simulink model "tau_7_1"  (R2019b)
settings: Solver=VariableStepAuto  StartTime=0.0  StopTime=9  RelTol=1e-3
model workspace (MAT data in the model file):
  k = 0.5
libraries: slctrlblks x10, simulink x5
settings Model: Creator=Sergey  LastModifiedBy=Sergey

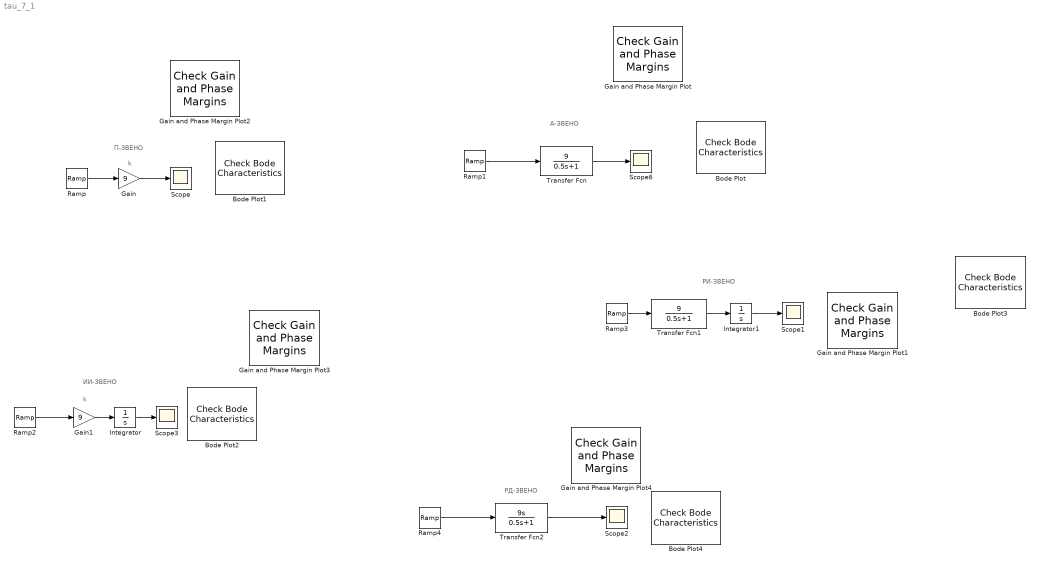
== system tau_7_1 ==
  note: РД-ЗВЕНО
  note: РИ-ЗВЕНО
  note: ИИ-ЗВЕНО
  note: А-ЗВЕНО
  note: П-ЗВЕНО
  note: k
  note: k
  Bode Plot : slctrlblks/Model Verification/Check Bode  Characteristics  InstantiateOnLoad=on  SaveOperatingPoints=off  LinearizationIOs={'/Ramp1', 1, 'in', 'off', '';'/Transfer Fcn', 1, 'out', 'off', ''}  LinearizeAt=SnapshotTimes  SnapshotTimes=[0]  TriggerType=rising  SampleTime=auto  RateConversionMethod=zoh  PreWarpFreq=10  UseExactDelayModel=off  UseFullBlockNameLabels=off  UseBusSignalLabels=off  enabled=on  stopWhenAssertionFail=off  export=off  ViewDlgPos=[1 41 1920 963]  OpenViewOnLoad=off  LaunchViewOnOpen=on  FrequencyUnits=rad/s  MagnitudeUnits=dB  PhaseUnits=deg  TimeUnits=seconds  EnableUpperBound=off  UpperBoundFrequencies=[]  UpperBoundMagnitudes=[]  EnableLowerBound=off  LowerBoundFrequencies=[]  LowerBoundMagnitudes=[]
      settings: SourceProductName=Simulink Control Design
  Bode Plot1 : slctrlblks/Model Verification/Check Bode  Characteristics  InstantiateOnLoad=on  SaveOperatingPoints=off  LinearizationIOs={'/Ramp', 1, 'in', 'off', '';'/Gain', 1, 'out', 'off', ''}  LinearizeAt=SnapshotTimes  SnapshotTimes=[0]  TriggerType=rising  SampleTime=auto  RateConversionMethod=zoh  PreWarpFreq=10  UseExactDelayModel=off  UseFullBlockNameLabels=off  UseBusSignalLabels=off  enabled=on  stopWhenAssertionFail=off  export=off  ViewDlgPos=[1 41 1920 963]  OpenViewOnLoad=off  LaunchViewOnOpen=on  FrequencyUnits=rad/s  MagnitudeUnits=dB  PhaseUnits=deg  TimeUnits=seconds  EnableUpperBound=off  UpperBoundFrequencies=[]  UpperBoundMagnitudes=[]  EnableLowerBound=off  LowerBoundFrequencies=[]  LowerBoundMagnitudes=[]
      settings: SourceProductName=Simulink Control Design
  Bode Plot2 : slctrlblks/Model Verification/Check Bode  Characteristics  InstantiateOnLoad=on  SaveOperatingPoints=off  LinearizationIOs={'/Ramp2', 1, 'in', 'off', '';'/Integrator', 1, 'out', 'off', ''}  LinearizeAt=SnapshotTimes  SnapshotTimes=[0]  TriggerType=rising  SampleTime=auto  RateConversionMethod=zoh  PreWarpFreq=10  UseExactDelayModel=off  UseFullBlockNameLabels=off  UseBusSignalLabels=off  enabled=on  stopWhenAssertionFail=off  export=off  ViewDlgPos=[1 41 1920 963]  OpenViewOnLoad=off  LaunchViewOnOpen=on  FrequencyUnits=rad/s  MagnitudeUnits=dB  PhaseUnits=deg  TimeUnits=seconds  EnableUpperBound=off  UpperBoundFrequencies=[]  UpperBoundMagnitudes=[]  EnableLowerBound=off  LowerBoundFrequencies=[]  LowerBoundMagnitudes=[]
      settings: SourceProductName=Simulink Control Design
  Bode Plot3 : slctrlblks/Model Verification/Check Bode  Characteristics  InstantiateOnLoad=on  SaveOperatingPoints=off  LinearizationIOs={'/Integrator1', 1, 'out', 'off', '';'/Ramp3', 1, 'in', 'off', ''}  LinearizeAt=SnapshotTimes  SnapshotTimes=[0]  TriggerType=rising  SampleTime=auto  RateConversionMethod=zoh  PreWarpFreq=10  UseExactDelayModel=off  UseFullBlockNameLabels=off  UseBusSignalLabels=off  enabled=on  stopWhenAssertionFail=off  export=off  ViewDlgPos=[1 41 1920 963]  OpenViewOnLoad=off  LaunchViewOnOpen=on  FrequencyUnits=rad/s  MagnitudeUnits=dB  PhaseUnits=deg  TimeUnits=seconds  EnableUpperBound=off  UpperBoundFrequencies=[]  UpperBoundMagnitudes=[]  EnableLowerBound=off  LowerBoundFrequencies=[]  LowerBoundMagnitudes=[]
      settings: SourceProductName=Simulink Control Design
  Bode Plot4 : slctrlblks/Model Verification/Check Bode  Characteristics  InstantiateOnLoad=on  SaveOperatingPoints=off  LinearizationIOs={'/Ramp4', 1, 'in', 'off', '';'/Transfer Fcn2', 1, 'out', 'off', ''}  LinearizeAt=SnapshotTimes  SnapshotTimes=[0]  TriggerType=rising  SampleTime=auto  RateConversionMethod=zoh  PreWarpFreq=10  UseExactDelayModel=off  UseFullBlockNameLabels=off  UseBusSignalLabels=off  enabled=on  stopWhenAssertionFail=off  export=off  ViewDlgPos=[1 41 1920 963]  OpenViewOnLoad=off  LaunchViewOnOpen=on  FrequencyUnits=rad/s  MagnitudeUnits=dB  PhaseUnits=deg  TimeUnits=seconds  EnableUpperBound=off  UpperBoundFrequencies=[]  UpperBoundMagnitudes=[]  EnableLowerBound=off  LowerBoundFrequencies=[]  LowerBoundMagnitudes=[]
      settings: SourceProductName=Simulink Control Design
  Gain : Gain  Gain=9
  Gain and Phase Margin Plot : slctrlblks/Model Verification/Check Gain and Phase Margins  InstantiateOnLoad=on  SaveOperatingPoints=off  LinearizationIOs={'/Ramp1', 1, 'in', 'off', '';'/Transfer Fcn', 1, 'out', 'off', ''}  LinearizeAt=SnapshotTimes  SnapshotTimes=[0]  TriggerType=rising  SampleTime=auto  RateConversionMethod=zoh  PreWarpFreq=10  UseExactDelayModel=off  UseFullBlockNameLabels=off  UseBusSignalLabels=off  enabled=on  stopWhenAssertionFail=off  export=off  ViewDlgPos=[1 41 1920 963]  LaunchViewOnOpen=on  OpenViewOnLoad=off  FrequencyUnits=rad/s  MagnitudeUnits=dB  PhaseUnits=deg  TimeUnits=seconds  EnableMargins=off  GainMargin=[]  PhaseMargin=[]  PlotType=nyquist  FeedbackSign=-1
      settings: SourceProductName=Simulink Control Design  SourceProductBaseCode=SD  SaveToWorkspace=off  SaveName=sys
  Gain and Phase Margin Plot1 : slctrlblks/Model Verification/Check Gain and Phase Margins  InstantiateOnLoad=on  SaveOperatingPoints=off  LinearizationIOs={'/Ramp3', 1, 'in', 'off', '';'/Integrator1', 1, 'out', 'off', ''}  LinearizeAt=SnapshotTimes  SnapshotTimes=[0]  TriggerType=rising  SampleTime=auto  RateConversionMethod=zoh  PreWarpFreq=10  UseExactDelayModel=off  UseFullBlockNameLabels=off  UseBusSignalLabels=off  enabled=on  stopWhenAssertionFail=off  export=off  ViewDlgPos=[1 41 1920 963]  LaunchViewOnOpen=on  OpenViewOnLoad=off  FrequencyUnits=rad/s  MagnitudeUnits=dB  PhaseUnits=deg  TimeUnits=seconds  EnableMargins=off  GainMargin=[]  PhaseMargin=[]  PlotType=nyquist  FeedbackSign=-1
      settings: SourceProductName=Simulink Control Design  SourceProductBaseCode=SD  SaveToWorkspace=off  SaveName=sys
  Gain and Phase Margin Plot2 : slctrlblks/Model Verification/Check Gain and Phase Margins  InstantiateOnLoad=on  SaveOperatingPoints=off  LinearizationIOs={'/Ramp', 1, 'in', 'off', '';'/Gain', 1, 'out', 'off', ''}  LinearizeAt=SnapshotTimes  SnapshotTimes=[0]  TriggerType=rising  SampleTime=auto  RateConversionMethod=zoh  PreWarpFreq=10  UseExactDelayModel=off  UseFullBlockNameLabels=off  UseBusSignalLabels=off  enabled=on  stopWhenAssertionFail=off  export=off  ViewDlgPos=[1 41 1920 963]  LaunchViewOnOpen=on  OpenViewOnLoad=off  FrequencyUnits=rad/s  MagnitudeUnits=dB  PhaseUnits=deg  TimeUnits=seconds  EnableMargins=off  GainMargin=[]  PhaseMargin=[]  PlotType=nyquist  FeedbackSign=-1
      settings: SourceProductName=Simulink Control Design  SourceProductBaseCode=SD  SaveToWorkspace=off  SaveName=sys
  Gain and Phase Margin Plot3 : slctrlblks/Model Verification/Check Gain and Phase Margins  InstantiateOnLoad=on  SaveOperatingPoints=off  LinearizationIOs={'/Ramp2', 1, 'in', 'off', '';'/Integrator', 1, 'out', 'off', ''}  LinearizeAt=SnapshotTimes  SnapshotTimes=[0]  TriggerType=rising  SampleTime=auto  RateConversionMethod=zoh  PreWarpFreq=10  UseExactDelayModel=off  UseFullBlockNameLabels=off  UseBusSignalLabels=off  enabled=on  stopWhenAssertionFail=off  export=off  ViewDlgPos=[1 41 1920 963]  LaunchViewOnOpen=on  OpenViewOnLoad=off  FrequencyUnits=rad/s  MagnitudeUnits=dB  PhaseUnits=deg  TimeUnits=seconds  EnableMargins=off  GainMargin=[]  PhaseMargin=[]  PlotType=nyquist  FeedbackSign=-1
      settings: SourceProductName=Simulink Control Design  SourceProductBaseCode=SD  SaveToWorkspace=off  SaveName=sys
  Gain and Phase Margin Plot4 : slctrlblks/Model Verification/Check Gain and Phase Margins  InstantiateOnLoad=on  SaveOperatingPoints=off  LinearizationIOs={'/Ramp4', 1, 'in', 'off', '';'/Transfer Fcn2', 1, 'out', 'off', ''}  LinearizeAt=SnapshotTimes  SnapshotTimes=[0]  TriggerType=rising  SampleTime=auto  RateConversionMethod=zoh  PreWarpFreq=10  UseExactDelayModel=off  UseFullBlockNameLabels=off  UseBusSignalLabels=off  enabled=on  stopWhenAssertionFail=off  export=off  ViewDlgPos=[1 41 1920 963]  LaunchViewOnOpen=on  OpenViewOnLoad=off  FrequencyUnits=rad/s  MagnitudeUnits=dB  PhaseUnits=deg  TimeUnits=seconds  EnableMargins=off  GainMargin=[]  PhaseMargin=[]  PlotType=nyquist  FeedbackSign=-1
      settings: SourceProductName=Simulink Control Design  SourceProductBaseCode=SD  SaveToWorkspace=off  SaveName=sys
  Gain1 : Gain  Gain=9
  Integrator : Integrator
  Integrator1 : Integrator
  Ramp{,1..4} (5 alike) : simulink/Sources/Ramp  slope=0  start=0  InitialOutput=1
  Scope{,1..3,6} (5 alike) : Scope
  Transfer Fcn : TransferFcn  Numerator=[9]  Denominator=[0.5 1]
  Transfer Fcn1 : TransferFcn  Numerator=[9]  Denominator=[0.5 1]
  Transfer Fcn2 : TransferFcn  Numerator=[9 0]  Denominator=[0.5 1]
  wires:
  Ramp/1 -> Gain/1
  Gain/1 -> Scope/1
  Ramp1/1 -> Transfer Fcn/1
  Transfer Fcn/1 -> Scope6/1
  Gain1/1 -> Integrator/1
  Ramp2/1 -> Gain1/1
  Transfer Fcn1/1 -> Integrator1/1
  Ramp3/1 -> Transfer Fcn1/1
  Integrator1/1 -> Scope1/1
  Ramp4/1 -> Transfer Fcn2/1
  Transfer Fcn2/1 -> Scope2/1
  Integrator/1 -> Scope3/1
